simulink model "barrier_template_14a"  (R2014a)
settings: Solver=ode3  StartTime=0.0  StopTime=inf  FixedStep=0.1  RelTol=1e-3
settings Model: CovSFcnEnable=on  Creator=gkovacs  LastModifiedBy=cloud
settings DataIOCC: SignalLoggingSaveFormat=ModelDataLogs
settings OptimizationCC: InitFltsAndDblsToZero=on
settings DebuggingCC: SaveWithParameterizedLinksMsg=none  UnderspecifiedInitializationDetection=Classic  SignalResolutionControl=TryResolveAllWithWarning  MultiTaskDSMMsg=warning  MultiTaskCondExecSysMsg=none  FcnCallInpInsideContextMsg=EnableAllAsWarning  FrameProcessingCompatibilityMsg=error
settings GRTTargetCC: TargetFcnLib=ansi_tfl_tmw.mat  GeneratePreprocessorConditionals=Use local settings  CombineOutputUpdateFcns=off  GRTInterface=on

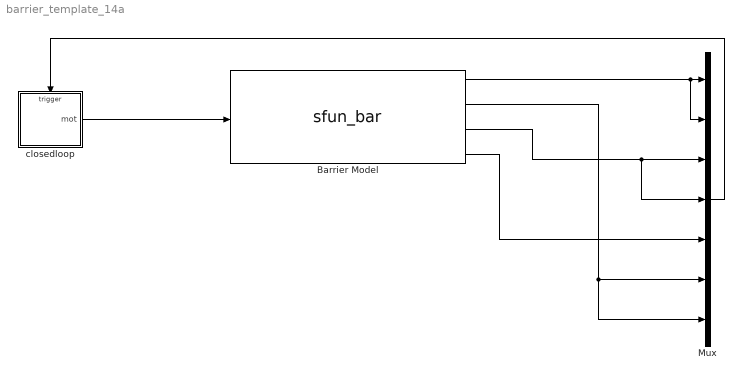
== system barrier_template_14a ==
  Barrier Model : M-S-Function  FunctionName=sfun_bar
      mask Display:
      | port_label('input',1,'Motor');
      | port_label('output',1,'Limit Switch Bottom');
      | port_label('output',2,'Limit Switch Top');
      | port_label('output',3,'IR');
      | port_label('output',4,'Remote');
      | text(0.05,0.9,'Barrier UI');
  Mux : Mux  Inputs=7
  closedloop : Stateflow chart  TreatAsAtomicUnit=on
      settings: PermitHierarchicalResolution=ParametersOnly
  wires:
  Barrier Model/1 -> Mux/2, Mux/1
  Barrier Model/2 -> Mux/6, Mux/7
  Barrier Model/3 -> Mux/4, Mux/3
  Barrier Model/4 -> Mux/5
  closedloop/1(mot) -> Barrier Model/1
  Mux/1 -> closedloop/Trigger

== stateflow chart barrier_template_14a/closedloop ==
  settings: executeAtInitialization=1
  state q0
  state q10
    entry:mot_d0;
    q10 -> q10 [order 1] : remote_rise
  state q11
    entry:mot_d0;
  state q12
    entry:mot_d0;
    q12 -> q12 [order 1] : remote_rise
  state q13
    entry:mot_d0;
  state q14
    entry:mot_d0;
    q14 -> q14 [order 1] : remote_rise
  state q15
    entry:mot_dm1;
    q15 -> q15 [order 1] : remote_rise
  state q16
    q16 -> q16 [order 1] : remote_rise
  state q17
    entry:mot_d1;
    q17 -> q17 [order 1] : remote_rise
  state q18
    entry:mot_d1;
    q18 -> q18 [order 1] : remote_rise
  state q19
    entry:mot_d0;
    q19 -> q19 [order 1] : remote_rise
  state q2
    entry:mot_d1;
    q2 -> q2 [order 1] : remote_rise
  state q20
    entry:mot_d0;
    q20 -> q20 [order 1] : remote_rise
  state q21
    q21 -> q21 [order 1] : remote_rise
  state q22
    q22 -> q22 [order 1] : remote_rise
  state q23
    q23 -> q23 [order 1] : remote_rise
  state q24
    q24 -> q24 [order 1] : remote_rise
  state q3
  state q4
    entry:mot_d1;
    q4 -> q4 [order 1] : remote_rise
  state q5
    entry:mot_d0;
    q5 -> q5 [order 1] : remote_rise
  state q6
  state q7
    entry:mot_d0;
    q7 -> q7 [order 1] : remote_rise
  state q8
    entry:mot_d0;
    q8 -> q8 [order 1] : remote_rise
  state q9
  q14 -> q12 [order 1] : infra_rise
  q11 -> q0 [order 1] : mot_d0/{mot=0;}
  q11 -> q13 [order 3] : infra_fall
  q8 -> q10 [order 1] : infra_fall
  q9 -> q11 [order 2] : bottom_rise
  q7 -> q10 [order 1] : top_fall
  (default) -> q0
  q12 -> q14 [order 1] : infra_fall
  q10 -> q18 [order 2] : mot_d0/{mot=0;}
  q0 -> q2 [order 1] : remote_rise
  q0 -> q3 [order 2] : infra_fall
  q12 -> q2 [order 2] : mot_d0/{mot=0;}
  q10 -> q8 [order 3] : infra_rise
  q13 -> q3 [order 3] : mot_d0/{mot=0;}
  q13 -> q14 [order 2] : remote_rise
  q3 -> q0 [order 1] : infra_rise
  q9 -> q10 [order 1] : infra_fall
  q10 -> q13 [order 1] : bottom_rise
  q13 -> q11 [order 1] : infra_rise
  q8 -> q11 [order 2] : bottom_rise
  q11 -> q12 [order 2] : remote_rise
  q8 -> q17 [order 3] : mot_d0/{mot=0;}
  q16 -> q15 [order 1] : infra_rise
  q19 -> q15 [order 1] : mot_d0/{mot=0;}
  q20 -> q16 [order 1] : mot_d0/{mot=0;}
  q17 -> q21 [order 2] : mot_d1/{mot=1;}
  q18 -> q22 [order 2] : mot_d1/{mot=1;}
  q15 -> q6 [order 2] : mot_dm1/{mot=-1;}
  q14 -> q4 [order 2] : mot_d0/{mot=0;}
  q23 -> q21 [order 1] : bottom_fall
  q24 -> q22 [order 1] : bottom_fall
  q22 -> q20 [order 1] : top_rise
  q5 -> q15 [order 1] : mot_d0/{mot=0;}
  q15 -> q16 [order 1] : infra_fall
  q7 -> q16 [order 2] : mot_d0/{mot=0;}
  q18 -> q17 [order 1] : infra_rise
  q17 -> q18 [order 1] : infra_fall
  q21 -> q22 [order 2] : infra_fall
  q2 -> q4 [order 2] : infra_fall
  q2 -> q23 [order 1] : mot_d1/{mot=1;}
  q7 -> q5 [order 3] : infra_rise
  q20 -> q19 [order 2] : infra_rise
  q21 -> q19 [order 1] : top_rise
  q19 -> q20 [order 2] : infra_fall
  q4 -> q2 [order 1] : infra_rise
  q22 -> q21 [order 2] : infra_rise
  q24 -> q23 [order 2] : infra_rise
  q6 -> q9 [order 3] : top_fall
  q5 -> q7 [order 2] : infra_fall
  q5 -> q8 [order 3] : top_fall
  q23 -> q24 [order 2] : infra_fall
  q6 -> q5 [order 1] : remote_rise
  q4 -> q24 [order 2] : mot_d1/{mot=1;}
  q3 -> q4 [order 2] : remote_rise
  q6 -> q7 [order 2] : infra_fall
  q9 -> q8 [order 3] : remote_rise
  data: mot output
  events: bottom_fall input FALLING_EDGE_EVENT; bottom_rise input RISING_EDGE_EVENT; infra_fall input FALLING_EDGE_EVENT; infra_rise input RISING_EDGE_EVENT; mot_d0 local FUNCTION_CALL_EVENT; mot_d1 local FUNCTION_CALL_EVENT; mot_dm1 local FUNCTION_CALL_EVENT; remote_rise input RISING_EDGE_EVENT; top_fall input FALLING_EDGE_EVENT; top_rise input RISING_EDGE_EVENT
